simulink model "lab_exer_mat_1"  (R2015a)
settings: Solver=ode45  StartTime=0.0  StopTime=inf  RelTol=1e-3
InitFcn:
  | CG_Init;
StopFcn:
  | CG_Stop;
values from neighbouring files (symbols this model uses):
  Ts = 1    [CG_Init.m]
settings Model: Creator=ees1504  LastModifiedBy=tamias
settings DataIOCC: SignalLoggingSaveFormat=ModelDataLogs
settings OptimizationCC: ExpressionDepthLimit=2147483647
settings DebuggingCC: UnderspecifiedInitializationDetection=Classic  MergeDetectMultiDrivingBlocksExec=none  SolverPrmCheckMsg=warning  StateNameClashWarn=warning
settings GRTTargetCC: CombineOutputUpdateFcns=off  GRTInterface=on

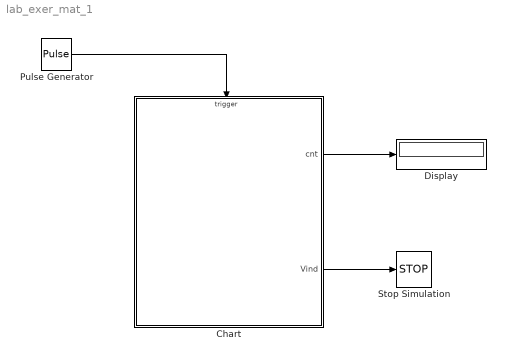
== system lab_exer_mat_1 ==
  Chart : Stateflow chart  TreatAsAtomicUnit=on
  Display : Display
  Pulse Generator : DiscretePulseGenerator  PulseType=Time based  Period=Ts  PulseWidth=0.5
  Stop Simulation : Stop
  wires:
  Chart/1(cnt) -> Display/1
  Chart/2(Vind) -> Stop Simulation/1
  Pulse Generator/1 -> Chart/Trigger

== stateflow chart lab_exer_mat_1/Chart ==
  state C [parallel]
    settings: executionOrder=1
    state UpCounter
      entry: upc = upc + 1;
      during: upc = upc + 1;
      UpCounter -> UpCounter
    (default) -> UpCounter : {upc=0;}
  state D [parallel]
    settings: executionOrder=2
    state S_end
      entry: Vind = 1;
    state S0
      entry: cnt = cnt + 1;
      ml.char_vals[cnt] = ml.randi(ml.Range, 1, 1);
      ml.time_vals[cnt] = upc;
    state S5
    state S4
    state S3
    state S2
    state S1
    (default) -> S0 : {cnt=0;Vind=0;}
    (junction 53) -> S_end [order 2] : [cnt==ml.Nc]
    S5 -> S0
    (junction 61) -> S0 [order 2] : [val<=ml.qs[3]]
    S0 -> (junction 53)
    (junction 28) -> S0 [order 1] : [val<=ml.qs[1]]
    (junction 34) -> S0 [order 2] : [val<=ml.qs[2]]
    S4 -> (junction 61) : {val=ml.rand(1);}
    (junction 61) -> S5 [order 1] : [val>ml.qs[3]]
    (junction 53) -> S1 [order 1] : [cnt!=ml.Nc]
    S3 -> S4
    (junction 34) -> S3 [order 1] : [val>ml.qs[2]]
    (junction 28) -> S2 [order 2] : [val>ml.qs[1]]
    S2 -> (junction 34) : {val=ml.rand(1);}
    S1 -> (junction 28) : {val=ml.rand(1);}
  data: val local double; cnt output double; Vind output boolean; upc local int32
  events: clk input RISING_EDGE_EVENT
